simulink model "Filter"  (R2020b)
settings: Solver=VariableStepAuto  StartTime=0.0  StopTime=10.0  RelTol=1e-3
settings Model: Creator=omkar  LastModifiedBy=omkar
settings DataIOCC: SaveOutput=off  SaveTime=off

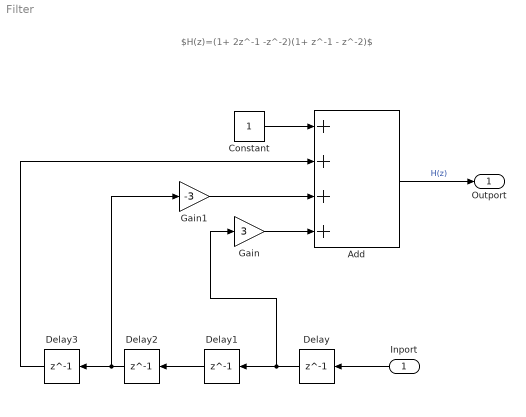
== system Filter ==
  note: $H(z)=(1+ 2z^-1 -z^-2)(1+ z^-1 - z^-2)$
  Inport : Inport
  Add : Sum  Inputs=++++
  Constant : Constant
  Delay{,1..3} (4 alike) : Delay  DelayLength=1
  Gain : Gain  Gain=3
  Gain1 : Gain  Gain=-3
  Outport : Outport  OutDataTypeStr=double  PortDimensions=1  SampleTime=[0.20000000000000001,0]
  wires:
  Delay1/1 -> Delay2/1
  Delay/1 -> Delay1/1, Gain/1
  Constant/1 -> Add/1
  Delay2/1 -> Delay3/1, Gain1/1
  Add/1 -> Outport/1  "H(z)"
  Gain/1 -> Add/4
  Inport/1 -> Delay/1
  Gain1/1 -> Add/3
  Delay3/1 -> Add/2
